simulink model "MultipleClockDelay"  (Simulink 6.3)
settings: Solver=FixedStepDiscrete  SolverMode=SingleTasking  StartTime=0.0  StopTime=1e-5  RelTol=1e-3
InitFcn:
  | %% DSPBuilder Start
  | alt_dspbuilder_update_model(bdroot)
  | %% DSPBuilder End
libraries: allblocks_alteradspbuilder2 x9
settings Model: LastModifiedBy=ascott  StrictBusMsg=None
settings DataIOCC: SignalLoggingName=sigsOut
settings OptimizationCC: BooleanDataType=off  InlineInvariantSignals=on
settings DebuggingCC: SolverPrmCheckMsg=none
settings HardwareCC: TargetUnknown=on

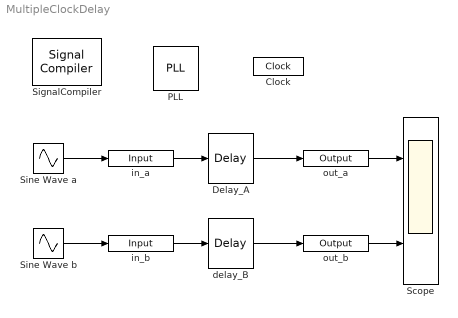
== system MultipleClockDelay ==
  Clock : allblocks_alteradspbuilder2/Clock  ClockPeriod=100  ClockPeriodUnit=ns  SampleTime=1e-007  SimulationStartCycle=5  PhaseOffset=0  Reset=aclr  ResetType=Active Low  Export=off
  Delay_A : allblocks_alteradspbuilder2/Delay  pipeline=1  ClockPhase=1  use_ena=off  use_sclr=off
  PLL : allblocks_alteradspbuilder2/PLL  clock_mult=[8, 1, 1, 1, 1, 1, 1, 1, 1]  clock_divide=[1, 1, 1, 1, 1, 1, 1, 1, 1]  clock_export=[0, 0, 0, 0, 0, 0, 0, 0, 0]  num_clocks=2  input_clock=Clock  use_base_clock=on
  Scope : Scope  NumInputPorts=2
      settings: YMin=-150~-150  YMax=150~150  SampleInput=on
  SignalCompiler : allblocks_alteradspbuilder2/Signal Compiler  DeviceFamily=Stratix III  DeviceName=AUTO  EnableSignalTap=off  SignalTapDepth=128  UseBoardBlock=off  StpUseDefaultClock=on  StpClock=Clock
  Sine Wave a : Sin  SineType=Sample based  Amplitude=2^7-1  Samples=20  SampleTime=8e-7
  Sine Wave b : Sin  SineType=Sample based  Amplitude=2^7-1  Samples=20  SampleTime=1e-7
  delay_B : allblocks_alteradspbuilder2/Delay  pipeline=1  ClockPhase=1  use_ena=off  use_sclr=off
  in_a : allblocks_alteradspbuilder2/Input  iofile=D:\eclipse_workspaces\DSPBuilder\Documentation\DesignExamples\Tutorials\MultiRate\Pll\tb_MultipleClockDelay\MultipleClockDelay_in_a.salt  BusType=Signed Integer  bwl=8  bwr=0  SpecifyClock=on  clock=PLL_clk0  PORTTYPE=Input
  in_b : allblocks_alteradspbuilder2/Input  iofile=D:\eclipse_workspaces\DSPBuilder\Documentation\DesignExamples\Tutorials\MultiRate\Pll\tb_MultipleClockDelay\MultipleClockDelay_in_b.salt  BusType=Signed Integer  bwl=8  bwr=0  SpecifyClock=on  clock=PLL_clk1  PORTTYPE=Input
  out_a : allblocks_alteradspbuilder2/Output  iofile=D:\eclipse_workspaces\DSPBuilder\Documentation\DesignExamples\Tutorials\MultiRate\Pll\tb_MultipleClockDelay\MultipleClockDelay_out_a.capture  BusType=Signed Integer  bwl=8  bwr=0  PORTTYPE=Output
  out_b : allblocks_alteradspbuilder2/Output  iofile=D:\eclipse_workspaces\DSPBuilder\Documentation\DesignExamples\Tutorials\MultiRate\Pll\tb_MultipleClockDelay\MultipleClockDelay_out_b.capture  BusType=Signed Integer  bwl=8  bwr=0  PORTTYPE=Output
  wires:
  in_a/1 -> Delay_A/1
  Delay_A/1 -> out_a/1
  delay_B/1 -> out_b/1
  in_b/1 -> delay_B/1
  Sine Wave a/1 -> in_a/1
  out_a/1 -> Scope/1
  out_b/1 -> Scope/2
  Sine Wave b/1 -> in_b/1
